simulink model "model_6ws6wd"  (R2023a)
settings: Solver=VariableStepAuto  StartTime=0.0  StopTime=20  RelTol=1e-3
settings Model: Creator=NGOC MAI  LastModifiedBy=NGOC MAI

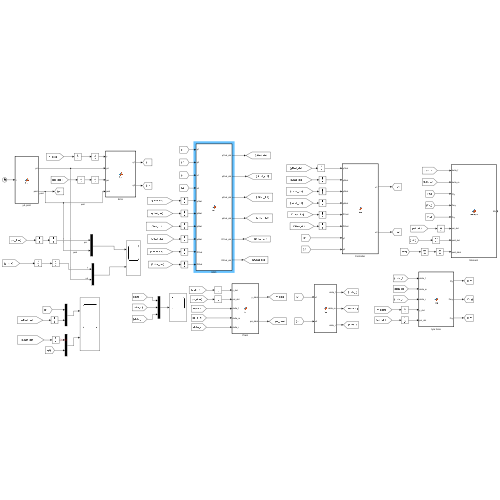
[thumbnail: Simulink's stored preview of the top-level diagram]
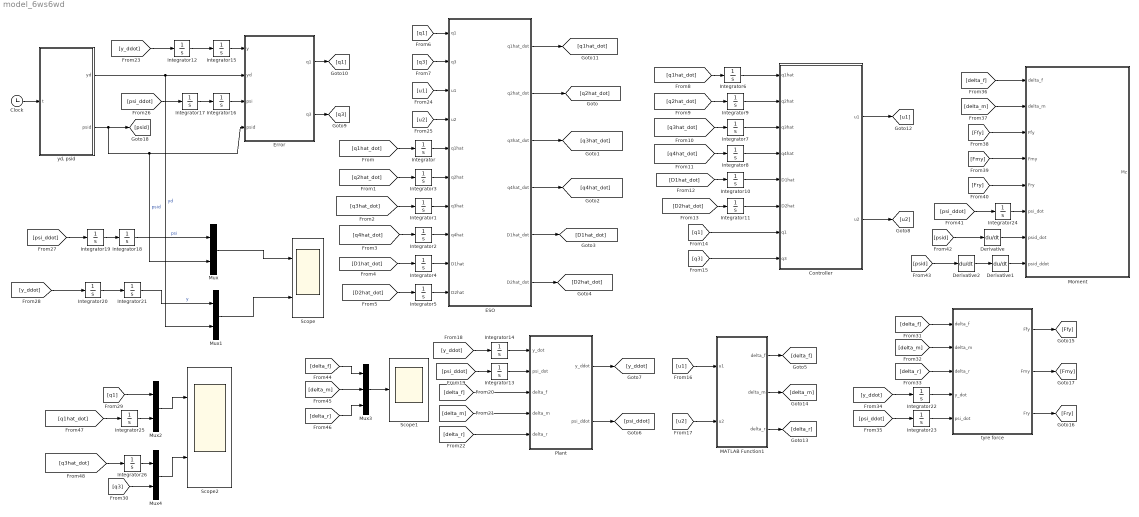
== system model_6ws6wd ==
  Clock : Clock
      settings: Decimation=20
  Controller : MATLAB Function  TreatAsAtomicUnit=on
  Derivative : Derivative
  Derivative1 : Derivative
  Derivative2 : Derivative
  ESO : MATLAB Function  TreatAsAtomicUnit=on
  Error : MATLAB Function  TreatAsAtomicUnit=on
  Integrator{,1..26} (27 alike) : Integrator
  MATLAB Function1 : MATLAB Function  TreatAsAtomicUnit=on
  Moment : MATLAB Function  TreatAsAtomicUnit=on
  Mux{,1..2,4} (4 alike) : Mux  Inputs=2
  Mux3 : Mux  Inputs=3
  Plant : MATLAB Function  TreatAsAtomicUnit=on
  Scope : Scope  NumInputPorts=2
  Scope1 : Scope
  Scope2 : Scope  NumInputPorts=2
  tyre force : MATLAB Function  TreatAsAtomicUnit=on
  "yd, psid" : MATLAB Function  TreatAsAtomicUnit=on
  wires:
  Clock/1 -> "yd, psid"/1(t)
  ESO/5(D1hat_dot) -> [D1hat_dot]
  ESO/6(D2hat_dot) -> [D2hat_dot]
  ESO/4(q4hat_dot) -> [q4hat_dot]
  ESO/3(q3hat_dot) -> [q3hat_dot]
  ESO/2(q2hat_dot) -> [q2hat_dot]
  ESO/1(q1hat_dot) -> [q1hat_dot]
  Integrator/1 -> ESO/5(q1hat)
  Integrator3/1 -> ESO/6(q2hat)
  Integrator1/1 -> ESO/7(q3hat)
  Integrator2/1 -> ESO/8(q4hat)
  [q1hat_dot] -> Integrator/1
  [q3hat_dot] -> Integrator1/1
  [q2hat_dot] -> Integrator3/1
  [q4hat_dot] -> Integrator2/1
  Integrator5/1 -> ESO/10(D2hat)
  Integrator4/1 -> ESO/9(D1hat)
  [D1hat_dot] -> Integrator4/1
  [D2hat_dot] -> Integrator5/1
  [q1] -> ESO/1(q1)
  [q3] -> ESO/2(q3)
  Error/2(q3) -> [q3]
  Error/1(q1) -> [q1]
  "yd, psid"/1(yd) -> Error/2(yd), Mux1/2  "yd"
  [q3hat_dot] -> Integrator7/1
  Integrator11/1 -> Controller/6(D2hat)
  Integrator6/1 -> Controller/1(q1hat)
  [D1hat_dot] -> Integrator10/1
  [q4hat_dot] -> Integrator8/1
  Integrator10/1 -> Controller/5(D1hat)
  Integrator7/1 -> Controller/3(q3hat)
  Integrator8/1 -> Controller/4(q4hat)
  [q1hat_dot] -> Integrator6/1
  [D2hat_dot] -> Integrator11/1
  [q2hat_dot] -> Integrator9/1
  Integrator9/1 -> Controller/2(q2hat)
  [q1] -> Controller/7(q1)
  [q3] -> Controller/8(q3)
  Controller/1(u1) -> [u1]
  Controller/2(u2) -> [u2]
  [u1] -> MATLAB Function1/1(u1)
  [u2] -> MATLAB Function1/2(u2)
  Integrator14/1 -> Plant/1(y_dot)
  [y_ddot] -> Integrator14/1
  [psi_ddot] -> Integrator13/1
  Integrator13/1 -> Plant/2(psi_dot)
  Plant/1(y_ddot) -> [y_ddot]
  Plant/2(psi_ddot) -> [psi_ddot]
  MATLAB Function1/1(delta_f) -> [delta_f]
  MATLAB Function1/2(delta_m) -> [delta_m]
  MATLAB Function1/3(delta_r) -> [delta_r]
  [delta_f] -> Plant/3(delta_f)
  [delta_m] -> Plant/4(delta_m)
  [delta_r] -> Plant/5(delta_r)
  [y_ddot] -> Integrator12/1
  Integrator12/1 -> Integrator15/1
  Integrator15/1 -> Error/1(y)
  [u1] -> ESO/3(u1)
  [u2] -> ESO/4(u2)
  [psi_ddot] -> Integrator17/1
  Integrator17/1 -> Integrator16/1
  Integrator16/1 -> Error/3(psi)
  [psi_ddot] -> Integrator19/1
  Integrator19/1 -> Integrator18/1
  Integrator20/1 -> Integrator21/1
  [y_ddot] -> Integrator20/1
  Integrator18/1 -> Mux/1  "psi"
  Integrator21/1 -> Mux1/1  "y"
  Mux/1 -> Scope/1
  Mux1/1 -> Scope/2
  [q1] -> Mux2/1
  [delta_f] -> tyre force/1(delta_f)
  [delta_m] -> tyre force/2(delta_m)
  [delta_r] -> tyre force/3(delta_r)
  Integrator22/1 -> tyre force/4(y_dot)
  Integrator23/1 -> tyre force/5(psi_dot)
  [y_ddot] -> Integrator22/1
  [psi_ddot] -> Integrator23/1
  [delta_f] -> Moment/1(delta_f)
  [delta_m] -> Moment/2(delta_m)
  tyre force/1(Ffy) -> [Ffy]
  tyre force/2(Fmy) -> [Fmy]
  tyre force/3(Fry) -> [Fry]
  [Ffy] -> Moment/3(Ffy)
  [Fmy] -> Moment/4(Fmy)
  [Fry] -> Moment/5(Fry)
  [psi_ddot] -> Integrator24/1
  Integrator24/1 -> Moment/6(psi_dot)
  "yd, psid"/2(psid) -> [psid], Mux/2, Error/4(psid)  "psid"
  [psid] -> Derivative/1
  Derivative/1 -> Moment/7(psid_dot)
  Derivative2/1 -> Derivative1/1
  Derivative1/1 -> Moment/8(psid_ddot)
  [psid] -> Derivative2/1
  [delta_f] -> Mux3/1
  [delta_m] -> Mux3/2
  [delta_r] -> Mux3/3
  Mux3/1 -> Scope1/1
  [q3] -> Mux4/2
  Integrator25/1 -> Mux2/2
  [q1hat_dot] -> Integrator25/1
  Mux2/1 -> Scope2/1
  [q3hat_dot] -> Integrator26/1
  ? -> ?
  Mux4/1 -> Scope2/2
  Integrator26/1 -> Mux4/1

== matlab function model_6ws6wd/tyre force ==
  data: Ffy output; delta_f input; delta_m input; delta_r input; y_dot input; psi_dot input; Fmy output; Fry output
function [Ffy,Fmy,Fry] = fcn(delta_f,delta_m,delta_r,y_dot,psi_dot)
cf=55000; %N/rad
cm=100000; %N/rad
cr=120000; %N/rad
lf=1.95; %m
lm=0.1; %m
lr=1.95; %m
vx=20; %m/s
Ffy=2*cf*(delta_f-(y_dot+lf*psi_dot)/vx);
Fmy=2*cm*(delta_m-(y_dot+lm*psi_dot)/vx);
Fry=2*cr*(delta_r-(y_dot-lr*psi_dot)/vx);
end

== matlab function model_6ws6wd/Error ==
  data: y input; q1 output; yd input; psi input; psid input; q3 output
function [q1,q3]= fcn(y,yd,psi,psid)
q1=y-yd;
q3=psi-psid;
end

== matlab function model_6ws6wd/Plant ==
  data: y_dot input; y_ddot output; psi_dot input; delta_f input; delta_m input; psi_ddot output; delta_r input
function [y_ddot,psi_ddot] = fcn(y_dot,psi_dot,delta_f,delta_m,delta_r)
m=8800; %kg
J=1350; %kgm^2
cf=55000; %N/rad
cm=100000; %N/rad
cr=120000; %N/rad
lf=1.95; %m
lm=0.1; %m
lr=1.95; %m
vx=20; %m/s
k1=(-2*cf-2*cr-2*cm)/(m*vx);
k2=2*(lf*cf+lr*cr+lm*cm)/(m*vx)-vx;
k3=2*(-lf*cf+lr*cr-lm*cm)/(J*vx);
k4=2*((lf^2)*cf-(lr^2)*cr+(lm^2)*cm)/(J*vx);
d1=9.8*cos(10);
u1=2*(cf*delta_f+cm*delta_m+cr*delta_r)/m;
u2=2*(lf*cf*delta_f+lm*cm*delta_m-lr*cr*delta_r)/J;
y_ddot=k1*y_dot+k2*psi_dot+u1+d1;
psi_ddot=k3*y_dot+k4*psi_dot+u2;
end

== matlab function model_6ws6wd/ESO ==
  data: q1 input; q1hat_dot output; q3 input; u1 input; u2 input; q1hat input; q2hat input; q3hat input; q4hat input; D1hat input; D2hat input; q2hat_dot output; q3hat_dot output; q4hat_dot output; D1hat_dot output; D2hat_dot output
function [q1hat_dot,q2hat_dot,q3hat_dot,q4hat_dot,D1hat_dot,D2hat_dot]= fcn(q1,q3,u1,u2,q1hat,q2hat,q3hat,q4hat,D1hat,D2hat)
m=8800; %kg
J=1350; %kgm^2
cf=55000; %N/rad
cm=100000; %N/rad
cr=120000; %N/rad
lf=1.95; %m
lm=0.1; %m
lr=1.95; %m
vx=20; %m/s

m1=2*(-cf-cr-cm)/(m*vx);
m2=2*(cf+cr+cm)/m;
m3=2*(lf*cf+lr*cr+lm*cm)/(m*vx);
n1=2*(-lf*cf+lr*cr-lm*cm)/(J*vx);
n2=2*(lf*cf-lr*cr+lm*cm)/J;
n3=2*((lf^2)*cf+(lm^2)*cm-(lr^2)*cr)/(J*vx);
a1=6;
a2=11;
a3=6;
epsi1=0.027;
epsi2=0.01;

q1hat_dot=q2hat+a1*(q1-q1hat)/epsi1;
q2hat_dot=D1hat+m1*q2hat+m2*q3hat+m3*q4hat+u1+a2*(q1-q1hat)/(epsi1^2);
D1hat_dot=a3*(q1-q1hat)/(epsi1^3);
q3hat_dot=q4hat+a1*(q3-q3hat)/epsi2;
q4hat_dot=D2hat+n1*q2hat+n2*q3hat+n3*q4hat+u2+a2*(q3-q3hat)/(epsi2^2);
D2hat_dot=a3*(q3-q3hat)/epsi2^3;
end

== matlab function model_6ws6wd/yd, psid ==
  data: t input; yd output; psid output
function [yd,psid]= fcn(t)
%yd=10*(tanh(3*t-35)-tanh(3*t-6));
%psid=(sech(3*t-60))^2-(sech(3*t-35)^2);
yd = 1.5*(tanh(t-6) - tanh(t-14));
psid = 1.5*(-(sech(t-14))^2 + (sech(t-6))^2)/20;
end

== matlab function model_6ws6wd/Controller ==
  data: u1 output; u2 output; q1hat input; q2hat input; q3hat input; q4hat input; D1hat input; D2hat input; q1 input; q3 input
function [u1, u2]= fcn(q1hat,q2hat,q3hat,q4hat,D1hat,D2hat,q1,q3)
%a1=6;
a2=11;
%a3=6;
epsi1=0.027;
epsi2=0.01;
p1=12;
p2=25;
c1=3;
c2=0.5;
c3=2;
c4=4;

m=8800; %kg
J=1350; %kgm^2
cf=55000; %N/rad
cm=100000; %N/rad
cr=120000; %N/rad
lf=1.95; %m
lm=0.1; %m
lr=1.95; %m
vx=20; %m/s

m1=2*(-cf-cr-cm)/(m*vx);
m2=2*(cf+cr+cm)/m;
m3=2*(lf*cf+lr*cr+lm*cm)/(m*vx);
%D1=9.8*cos(10)+m4*psid_dot+3*sin(t)+cos(t/2);
n1=2*(-lf*cf+lr*cr-lm*cm)/(J*vx);
n2=2*(lf*cf-lr*cr+lm*cm)/J;
n3=2*((lf^2)*cf+(lm^2)*cm-(lr^2)*cr)/(J*vx);
s1=p1*q1hat+q2hat;
s2=p2*q3hat+q4hat;

u1=-c1*s1-c2*sat(s1)-p1*q2hat-D1hat-m1*q2hat-m2*q3hat-m3*q4hat-a2*(q1-q1hat)/epsi1^2;
u2=-c3*s2-c4*sat(s2)-p2*q4hat-D2hat-n1*q2hat-n2*q3hat-n3*q4hat-a2*(q3-q3hat)/epsi2^2;
end

== matlab function model_6ws6wd/MATLAB Function1 ==
  data: u1 input; delta_f output; u2 input; delta_m output; delta_r output
function [delta_f,delta_m,delta_r] = fcn(u1,u2)
m=8800; %kg
J=1350; %kgm^2
cf=55000; %N/rad
cm=100000; %N/rad
cr=120000; %N/rad
lf=1.95; %m
lm=0.1; %m
lr=1.95; %m
%vx=20; %m/s
A=[cf cm cr;cf*lf cm*lm -cr*lr;1/2 -1 1/2];
B=[u1*m/2;u2*J/2;0];
C=A^(-1)*B;
delta_f=C(1,1);
delta_m=C(2,1);
delta_r=C(3,1);
end

== matlab function model_6ws6wd/Moment ==
  data: delta_f input; Mz output; delta_m input; Ffy input; Fmy input; Fry input; psi_dot input; psid_dot input; psid_ddot input
function Mz = moment(delta_f,delta_m,Ffy,Fmy,Fry,psi_dot,psid_dot,psid_ddot)
lf=1.95; %m
lm=0.1; %m
lr=1.95; %m
J=1350; %kgm^2
k_slid=2;
s=psi_dot-psid_dot;
Mz=-2*lf*Ffy*cos(delta_f)-2*lm*Fmy*cos(delta_m)+2*lr*Fry+J*psid_ddot+J*k_slid*sat(s);
end
